simulink model "GolfSwing3D_KineticallyDrivenBlockCountStrip"  (R2024b)
settings: Solver=VariableStepAuto  StartTime=0.0  StopTime=StopTime  MaxStep=0.001  RelTol=1e-3
model workspace: external: MAT-File 3DModelInputs.mat (data not in the file)
undefined symbols (not defined in the file or in its folder): GripStrength, KillswitchFinalValue, KillswitchInitialValue, KillswitchStepTime, LeftLowerArmLength, PlaneTilt, RightLowerArmLength, UpperTorsoLength, X, Y, Z
libraries: nesl_utility x361, sm_lib x136, matrix_library x11, fl_lib x2, simulink x1
(part 11 of 13)

== matlab function GolfSwing3D_KineticallyDrivenBlockCountStrip/LScap Input Function/LScap Torque ==
  data: Time input; Killswitch input; JointTorqueLScapX output; LScapInputXA parameter; LScapInputYA parameter; LScapInputXB parameter; LScapInputYB parameter; LScapPositionSetpointX parameter; GlobalGain parameter; LScapConstantX parameter; JointTorqueLScapY output; LScapPositionInputX output; LScapPositionInputY output; LScapVelocityInputX output; LScapConstantY parameter; LScapTimeGainX parameter; LScapTimeGainY parameter; LScapInputXC parameter; LScapInputYC parameter; LScapPositionGainX parameter; LScapPositionGainY parameter; TargetLScapPositionX parameter; ModelingMode parameter; GlobalPCGain parameter; GlobalVCGain parameter; DampeningGlobalGain parameter; TargetImpactTime parameter; LScapAoX parameter; LScapAoY parameter; KinematicMode parameter; LScapDampeningX parameter; LScapDampeningY parameter; LScapPositionSetpointY parameter; LScapStartPositionX parameter; LScapStartPositionY parameter; LScapStartVelocityX parameter; LScapStartVelocityY parameter; LScapVCGainX parameter; LScapVCGainY parameter; LScapVelocityInputY output; LScapAccelerationInputX output; LScapAccelerationInputY output; LScapPCGainX parameter; LScapPCGainY parameter; LScapPositionX input; LScapPositionY input; LScapVelocityX input; LScapVelocityY input; ZVCFLScapTorqueX parameter; ZVCFLScapTorqueY parameter; TargetLScapPositionY parameter; TargetLScapVelocityX parameter; TargetLScapVelocityY parameter; LScapAfX parameter; LScapAfY parameter; LScapInputXD parameter; LScapInputXE parameter; LScapInputXF parameter; LScapInputXG parameter; LScapInputYD parameter; LScapInputYE parameter; LScapInputYF parameter; LScapInputYG parameter
function [JointTorqueLScapX,JointTorqueLScapY,LScapPositionInputX, LScapPositionInputY, LScapVelocityInputX,LScapVelocityInputY,LScapAccelerationInputX,LScapAccelerationInputY] = fcn(Time,Killswitch, LScapInputXA,LScapInputYA, LScapInputXB,LScapInputYB, LScapPositionSetpointX,GlobalGain,...
    LScapConstantX, LScapConstantY, LScapTimeGainX, LScapTimeGainY,...
    LScapInputXC, LScapInputYC, LScapPositionGainX, LScapPositionGainY,...
    TargetLScapPositionX, ModelingMode,GlobalPCGain, GlobalVCGain,DampeningGlobalGain,TargetImpactTime,LScapAoX, LScapAoY, KinematicMode, LScapDampeningX, LScapDampeningY, LScapPositionSetpointY, LScapStartPositionX,...
    LScapStartPositionY, LScapStartVelocityX, LScapStartVelocityY, LScapVCGainX,...
    LScapVCGainY, LScapPCGainX, LScapPCGainY, LScapPositionX, LScapPositionY, LScapVelocityX,...
    LScapVelocityY, ZVCFLScapTorqueX, ZVCFLScapTorqueY, TargetLScapPositionY, TargetLScapVelocityX,...
    TargetLScapVelocityY,LScapAfX, LScapAfY,LScapInputXD, LScapInputXE, LScapInputXF, LScapInputXG,...
LScapInputYD, LScapInputYE, LScapInputYF, LScapInputYG)

%Tau=Time/TargetImpactTime;
t=Time;

% %%%%%%%%%%%%%%%%%%%%%%%%%%%%%%%%%%%%%%%%%%%
% % Kinetic Input Selection and Calculation
% %%%%%%%%%%%%%%%%%%%%%%%%%%%%%%%%%%%%%%%%%%%

if ModelingMode==0
    % Values are all set to zero.
    JointTorqueLScapX=0;
    JointTorqueLScapY=0;
elseif ModelingMode==1
    % Control based strategy. Values are based on difference in value
    % between the current state and desired state.
    % LScap Joint Rotational Deltas
    DeltaLScapPositionX=LScapPositionX-TargetLScapPositionX;
    DeltaLScapPositionY=LScapPositionY-TargetLScapPositionY;
    DeltaLScapVelocityX=LScapVelocityX-TargetLScapVelocityX;
    DeltaLScapVelocityY=LScapVelocityY-TargetLScapVelocityY;
    % Control Based Strategy
    JointTorqueLScapX=DeltaLScapPositionX*LScapPCGainX*GlobalPCGain-DeltaLScapVelocityX*LScapVCGainX*GlobalVCGain-DampeningGlobalGain*LScapDampeningX*LScapVelocityX;
    JointTorqueLScapY=DeltaLScapPositionY*LScapPCGainY*GlobalPCGain-DeltaLScapVelocityY*LScapVCGainY*GlobalVCGain-DampeningGlobalGain*LScapDampeningY*LScapVelocityY;
elseif ModelingMode==2
    % Forward Dynamics Based Strategy. Values are computed based on a
    % polynomial and a combination of dampening and position gained
    % factors.
    JointTorqueLScapX=Killswitch*GlobalGain*(LScapConstantX+LScapTimeGainX*Time-LScapPositionGainX*(LScapPositionX-LScapPositionSetpointX)...
    -LScapDampeningX*LScapVelocityX);
    JointTorqueLScapY=Killswitch*GlobalGain*(LScapConstantY+LScapTimeGainY*Time-LScapPositionGainY*(LScapPositionY-LScapPositionSetpointY)...
    -LScapDampeningY*LScapVelocityY);
elseif ModelingMode==3
    JointTorqueLScapX=HexPolyInputFunction(LScapInputXA,LScapInputXB,LScapInputXC,LScapInputXD,LScapInputXE,LScapInputXF,LScapInputXG,Time)*Killswitch;
    JointTorqueLScapY=HexPolyInputFunction(LScapInputYA,LScapInputYB,LScapInputYC,LScapInputYD,LScapInputYE,LScapInputYF,LScapInputYG,Time)*Killswitch; 
else
    %ZVCF Based Joint Torques. Values are pulled from model workspace and
    %held constant.
    JointTorqueLScapX=ZVCFLScapTorqueX;
    JointTorqueLScapY=ZVCFLScapTorqueY;
end

% %%%%%%%%%%%%%%%%%%%%%%%%%%%%%%%%%%%%%%%%%%%
% % Kinematic Input Selection and Calculation
% %%%%%%%%%%%%%%%%%%%%%%%%%%%%%%%%%%%%%%%%%%%

if KinematicMode==0
    % All kinematic values set to zero.
    LScapPositionInputX=0;
    LScapPositionInputY=0;
    LScapVelocityInputX=0;
    LScapVelocityInputY=0;
    LScapAccelerationInputX=0;
    LScapAccelerationInputY=0;
elseif KinematicMode==1
    % 1st Order Acceleration, 2nd Order Velocity, 3rd Order Position Solution
    PTX=TargetLScapPositionX;       
    VTX=TargetLScapVelocityX;
    PTY=TargetLScapPositionY;
    VTY=TargetLScapVelocityY;
    % Define Starting Position and Velocity
    PIX=LScapStartPositionX;
    VIX=LScapStartVelocityX;
    PIY=LScapStartPositionY;
    VIY=LScapStartVelocityY;
    AX=3*((VTX+VIX)*TargetImpactTime-2*(PTX-PIX))/TargetImpactTime^3;         % Constant in position equation
    BX=-2*((VTX+2*VIX)*TargetImpactTime-3*(PTX-PIX))/TargetImpactTime^2;         % Constant in position equation
    CX=VIX;         % Starting Velocity at Time Zero
    DX=PIX;         % Starting Position at Time Zero
    AY=3*((VTY+VIY)*TargetImpactTime-2*(PTY-PIY))/TargetImpactTime^3;         % Constant in position equation
    BY=-2*((VTY+2*VIY)*TargetImpactTime-3*(PTY-PIY))/TargetImpactTime^2;         % Constant in position equation
    CY=VIY;         % Starting Velocity at Time Zero
    DY=PIY;         % Starting Position at Time Zero
    % Equation for position as a function of time
    LScapPositionInputX=AX*Time^3/3+BX*Time^2/2+CX*Time+DX;
    LScapPositionInputY=AY*Time^3/3+BY*Time^2/2+CY*Time+DY;
    LScapVelocityInputX=AX*Time^2+BX*Time+CX;
    LScapVelocityInputY=AY*Time^2+BY*Time+CY;
    LScapAccelerationInputX=2*AX*Time+BX;
    LScapAccelerationInputY=2*AY*Time+BY;
elseif KinematicMode==2
    % 2nd Order Acceleration, 3rd Order Velocity, 4th Order Position Solution
    Tt=TargetImpactTime;
    t=Time;
    PoX=LScapStartPositionX;
    PoY=LScapStartPositionY;
    VoX=LScapStartVelocityX;
    VoY=LScapStartVelocityY;
    PfX=TargetLScapPositionX;
    PfY=TargetLScapPositionY;
    VfX=TargetLScapVelocityX;
    VfY=TargetLScapVelocityY;
    AoX=LScapAoX;
    AoY=LScapAoY;
    LScapPositionInputX=PoX + VoX*t + (AoX*t^2)/2 - (t^3*(4*PoX - 4*PfX + Tt*VfX + 3*Tt*VoX + AoX*Tt^2))/Tt^3 + (t^4*(6*PoX - 6*PfX + 2*Tt*VfX + 4*Tt*VoX + AoX*Tt^2))/(2*Tt^4);
    LScapPositionInputY=PoY + VoY*t + (AoY*t^2)/2 - (t^3*(4*PoY - 4*PfY + Tt*VfY + 3*Tt*VoY + AoY*Tt^2))/Tt^3 + (t^4*(6*PoY - 6*PfY + 2*Tt*VfY + 4*Tt*VoY + AoY*Tt^2))/(2*Tt^4);
    LScapVelocityInputX=VoX + AoX*t - (3*t^2*(4*PoX - 4*PfX + Tt*VfX + 3*Tt*VoX + AoX*Tt^2))/Tt^3 + (2*t^3*(6*PoX - 6*PfX + 2*Tt*VfX + 4*Tt*VoX + AoX*Tt^2))/Tt^4;
    LScapVelocityInputY=VoY + AoY*t - (3*t^2*(4*PoY - 4*PfY + Tt*VfY + 3*Tt*VoY + AoY*Tt^2))/Tt^3 + (2*t^3*(6*PoY - 6*PfY + 2*Tt*VfY + 4*Tt*VoY + AoY*Tt^2))/Tt^4;
    LScapAccelerationInputX=AoX + (6*t^2*(6*PoX - 6*PfX + 2*Tt*VfX + 4*Tt*VoX + AoX*Tt^2))/Tt^4 - (6*t*(4*PoX - 4*PfX + Tt*VfX + 3*Tt*VoX + AoX*Tt^2))/Tt^3;
    LScapAccelerationInputY=AoY + (6*t^2*(6*PoY - 6*PfY + 2*Tt*VfY + 4*Tt*VoY + AoY*Tt^2))/Tt^4 - (6*t*(4*PoY - 4*PfY + Tt*VfY + 3*Tt*VoY + AoY*Tt^2))/Tt^3;
else
    % 3rd Order Acceleration, 4th Order Velocity, 5th Order Position Solution
    Tt=TargetImpactTime;
    t=Time;
    PoX=LScapStartPositionX;
    PoY=LScapStartPositionY;
    VoX=LScapStartVelocityX;
    VoY=LScapStartVelocityY;
    PfX=TargetLScapPositionX;
    PfY=TargetLScapPositionY;
    VfX=TargetLScapVelocityX;
    VfY=TargetLScapVelocityY;
    AoX=LScapAoX;
    AoY=LScapAoY;
    AfX=LScapAfX;
    AfY=LScapAfY;
    LScapPositionInputX=PoX+VoX*t+(AoX*t^2)/2-(t^5*(12*PoX-12*PfX+6*Tt*VfX+6*Tt*VoX-AfX*Tt^2+AoX*Tt^2))/(2*Tt^5)-(t^3*(20*PoX-20*PfX+8*Tt*VfX+12*Tt*VoX-AfX*Tt^2+3*AoX*Tt^2))/(2*Tt^3)+(t^4*(30*PoX-30*PfX+14*Tt*VfX+16*Tt*VoX-2*AfX*Tt^2+3*AoX*Tt^2))/(2*Tt^4);
    LScapPositionInputY=PoY+VoY*t+(AoY*t^2)/2-(t^5*(12*PoY-12*PfY+6*Tt*VfY+6*Tt*VoY-AfY*Tt^2+AoY*Tt^2))/(2*Tt^5)-(t^3*(20*PoY-20*PfY+8*Tt*VfY+12*Tt*VoY-AfY*Tt^2+3*AoY*Tt^2))/(2*Tt^3)+(t^4*(30*PoY-30*PfY+14*Tt*VfY+16*Tt*VoY-2*AfY*Tt^2+3*AoY*Tt^2))/(2*Tt^4);  
    LScapVelocityInputX=VoX+AoX*t-(5*t^4*(12*PoX-12*PfX+6*Tt*VfX+6*Tt*VoX-AfX*Tt^2+AoX*Tt^2))/(2*Tt^5)-(3*t^2*(20*PoX-20*PfX+8*Tt*VfX+12*Tt*VoX-AfX*Tt^2+3*AoX*Tt^2))/(2*Tt^3)+(2*t^3*(30*PoX-30*PfX+14*Tt*VfX+16*Tt*VoX-2*AfX*Tt^2+3*AoX*Tt^2))/Tt^4;
    LScapVelocityInputY=VoY+AoY*t-(5*t^4*(12*PoY-12*PfY+6*Tt*VfY+6*Tt*VoY-AfY*Tt^2+AoY*Tt^2))/(2*Tt^5)-(3*t^2*(20*PoY-20*PfY+8*Tt*VfY+12*Tt*VoY-AfY*Tt^2+3*AoY*Tt^2))/(2*Tt^3)+(2*t^3*(30*PoY-30*PfY+14*Tt*VfY+16*Tt*VoY-2*AfY*Tt^2+3*AoY*Tt^2))/Tt^4;
    LScapAccelerationInputX=AoX-(3*t*(20*PoX-20*PfX+8*Tt*VfX+12*Tt*VoX-AfX*Tt^2+3*AoX*Tt^2))/Tt^3-(10*t^3*(12*PoX-12*PfX+6*Tt*VfX+6*Tt*VoX-AfX*Tt^2+AoX*Tt^2))/Tt^5+(6*t^2*(30*PoX-30*PfX+14*Tt*VfX+16*Tt*VoX-2*AfX*Tt^2+3*AoX*Tt^2))/Tt^4;
    LScapAccelerationInputY=AoY-(3*t*(20*PoY-20*PfY+8*Tt*VfY+12*Tt*VoY-AfY*Tt^2+3*AoY*Tt^2))/Tt^3-(10*t^3*(12*PoY-12*PfY+6*Tt*VfY+6*Tt*VoY-AfY*Tt^2+AoY*Tt^2))/Tt^5+(6*t^2*(30*PoY-30*PfY+14*Tt*VfY+16*Tt*VoY-2*AfY*Tt^2+3*AoY*Tt^2))/Tt^4;
end

% Calculate Higher Order Derivatives of the Position Outputs
LScapJerkX=gradient(LScapAccelerationInputX,t);
LScapJerkY=gradient(LScapAccelerationInputY,t);
LScapSnapX=gradient(LScapJerkX,t);
LScapSnapY=gradient(LScapJerkY,t);
LScapCrackleX=gradient(LScapSnapX,t);
LScapCrackleY=gradient(LScapSnapY,t);
LScapPopX=gradient(LScapCrackleX,t);
LScapPopY=gradient(LScapCrackleY,t);

== matlab function GolfSwing3D_KineticallyDrivenBlockCountStrip/RScap Input Function/RScap Torque ==
  data: Time input; Killswitch input; JointTorqueRScapX output; RScapInputXA parameter; RScapInputYA parameter; RScapInputXB parameter; RScapInputYB parameter; RScapPositionSetpointX parameter; GlobalGain parameter; RScapConstantX parameter; JointTorqueRScapY output; RScapConstantY parameter; RScapTimeGainX parameter; RScapTimeGainY parameter; RScapInputXC parameter; RScapInputYC parameter; RScapPositionGainX parameter; RScapPositionGainY parameter; TargetRScapPositionX parameter; ModelingMode parameter; GlobalPCGain parameter; GlobalVCGain parameter; DampeningGlobalGain parameter; TargetImpactTime parameter; KinematicMode parameter; RScapPositionSetpointY parameter; RScapStartPositionX parameter; RScapStartPositionY parameter; RScapVCGainX parameter; RScapVCGainY parameter; RScapPCGainX parameter; RScapPCGainY parameter; RScapPositionInputX output; RScapPositionInputY output; RScapVelocityInputX output; RScapVelocityInputY output; RScapAccelerationInputX output; RScapAccelerationInputY output; ZVCFRScapTorqueX parameter; ZVCFRScapTorqueY parameter; TargetRScapPositionY parameter; TargetRScapVelocityX parameter; TargetRScapVelocityY parameter; RScapAoX parameter; RScapAoY parameter; RScapDampeningX parameter; RScapDampeningY parameter; RScapPositionX input; RScapPositionY input; RScapVelocityX input; RScapVelocityY input; RScapStartVelocityX parameter; RScapStartVelocityY parameter; RScapAfX parameter; RScapAfY parameter; RScapInputXD parameter; RScapInputXE parameter; RScapInputXF parameter; RScapInputXG parameter; RScapInputYD parameter; RScapInputYE parameter; RScapInputYF parameter; RScapInputYG parameter
function [JointTorqueRScapX,JointTorqueRScapY,RScapPositionInputX,...
    RScapPositionInputY, RScapVelocityInputX,RScapVelocityInputY,...
    RScapAccelerationInputX,RScapAccelerationInputY] = fcn(Time,Killswitch,...
    RScapInputXA,RScapInputYA, RScapInputXB,RScapInputYB, RScapPositionSetpointX,GlobalGain,...
    RScapConstantX, RScapConstantY, RScapTimeGainX, RScapTimeGainY,...
    RScapInputXC, RScapInputYC, RScapPositionGainX, RScapPositionGainY,...
    TargetRScapPositionX, ModelingMode,GlobalPCGain, GlobalVCGain,DampeningGlobalGain,...
    TargetImpactTime,KinematicMode, RScapPositionSetpointY, RScapStartPositionX,...
    RScapStartPositionY, RScapVCGainX,RScapVCGainY, RScapPCGainX, RScapPCGainY,...
    ZVCFRScapTorqueX, ZVCFRScapTorqueY, ...
    TargetRScapPositionY, TargetRScapVelocityX, TargetRScapVelocityY,...
    RScapAoX, RScapAoY, RScapDampeningX, RScapDampeningY, RScapPositionX,...
    RScapPositionY, RScapVelocityX, RScapVelocityY, RScapStartVelocityX, RScapStartVelocityY,...
    RScapAfX, RScapAfY,RScapInputXD, RScapInputXE, RScapInputXF, RScapInputXG,...
RScapInputYD, RScapInputYE, RScapInputYF, RScapInputYG)

%Tau=Time/TargetImpactTime;
t=Time;

% %%%%%%%%%%%%%%%%%%%%%%%%%%%%%%%%%%%%%%%%%%%
% % Kinetic Input Selection and Calculation
% %%%%%%%%%%%%%%%%%%%%%%%%%%%%%%%%%%%%%%%%%%%

if ModelingMode==0
    % Values are all set to zero.
    JointTorqueRScapX=0;
    JointTorqueRScapY=0;
elseif ModelingMode==1
    % Control based strategy. Values are based on difference in value
    % between the current state and desired state.
    % RScap Joint Rotational Deltas
    DeltaRScapPositionX=RScapPositionX-TargetRScapPositionX;
    DeltaRScapPositionY=RScapPositionY-TargetRScapPositionY;
    DeltaRScapVelocityX=RScapVelocityX-TargetRScapVelocityX;
    DeltaRScapVelocityY=RScapVelocityY-TargetRScapVelocityY;
    % Control Based Strategy
    JointTorqueRScapX=DeltaRScapPositionX*RScapPCGainX*GlobalPCGain-DeltaRScapVelocityX*RScapVCGainX*GlobalVCGain-DampeningGlobalGain*RScapDampeningX*RScapVelocityX;
    JointTorqueRScapY=DeltaRScapPositionY*RScapPCGainY*GlobalPCGain-DeltaRScapVelocityY*RScapVCGainY*GlobalVCGain-DampeningGlobalGain*RScapDampeningY*RScapVelocityY;
elseif ModelingMode==2
    % Forward Dynamics Based Strategy. Values are computed based on a
    % polynomial and a combination of dampening and position gained
    % factors.
    JointTorqueRScapX=Killswitch*GlobalGain*(RScapConstantX+RScapTimeGainX*Time-RScapPositionGainX*(RScapPositionX-RScapPositionSetpointX)...
    -RScapDampeningX*RScapVelocityX);
    JointTorqueRScapY=Killswitch*GlobalGain*(RScapConstantY+RScapTimeGainY*Time-RScapPositionGainY*(RScapPositionY-RScapPositionSetpointY)...
    -RScapDampeningY*RScapVelocityY);
elseif ModelingMode==3
    JointTorqueRScapX=HexPolyInputFunction(RScapInputXA,RScapInputXB,RScapInputXC,RScapInputXD,RScapInputXE,RScapInputXF,RScapInputXG,Time)*Killswitch;
    JointTorqueRScapY=HexPolyInputFunction(RScapInputYA,RScapInputYB,RScapInputYC,RScapInputYD,RScapInputYE,RScapInputYF,RScapInputYG,Time)*Killswitch;  
else
    %ZVCF Based Joint Torques. Values are pulled from model workspace and
    %held constant.
    JointTorqueRScapX=ZVCFRScapTorqueX;
    JointTorqueRScapY=ZVCFRScapTorqueY;
end

% %%%%%%%%%%%%%%%%%%%%%%%%%%%%%%%%%%%%%%%%%%%
% % Kinematic Input Selection and Calculation
% %%%%%%%%%%%%%%%%%%%%%%%%%%%%%%%%%%%%%%%%%%%

if KinematicMode==0
    % All kinematic values set to zero.
    RScapPositionInputX=0;
    RScapPositionInputY=0;
    RScapVelocityInputX=0;
    RScapVelocityInputY=0;
    RScapAccelerationInputX=0;
    RScapAccelerationInputY=0;
elseif KinematicMode==1
    % 1st Order Acceleration, 2nd Order Velocity, 3rd Order Position Solution
    PTX=TargetRScapPositionX;       
    VTX=TargetRScapVelocityX;
    PTY=TargetRScapPositionY;
    VTY=TargetRScapVelocityY;
    % Define Starting Position and Velocity
    PIX=RScapStartPositionX;
    VIX=RScapStartVelocityX;
    PIY=RScapStartPositionY;
    VIY=RScapStartVelocityY;
    AX=3*((VTX+VIX)*TargetImpactTime-2*(PTX-PIX))/TargetImpactTime^3;         % Constant in position equation
    BX=-2*((VTX+2*VIX)*TargetImpactTime-3*(PTX-PIX))/TargetImpactTime^2;         % Constant in position equation
    CX=VIX;         % Starting Velocity at Time Zero
    DX=PIX;         % Starting Position at Time Zero
    AY=3*((VTY+VIY)*TargetImpactTime-2*(PTY-PIY))/TargetImpactTime^3;         % Constant in position equation
    BY=-2*((VTY+2*VIY)*TargetImpactTime-3*(PTY-PIY))/TargetImpactTime^2;         % Constant in position equation
    CY=VIY;         % Starting Velocity at Time Zero
    DY=PIY;         % Starting Position at Time Zero
    % Equation for position as a function of time
    RScapPositionInputX=AX*Time^3/3+BX*Time^2/2+CX*Time+DX;
    RScapPositionInputY=AY*Time^3/3+BY*Time^2/2+CY*Time+DY;
    RScapVelocityInputX=AX*Time^2+BX*Time+CX;
    RScapVelocityInputY=AY*Time^2+BY*Time+CY;
    RScapAccelerationInputX=2*AX*Time+BX;
    RScapAccelerationInputY=2*AY*Time+BY;
elseif KinematicMode==2
    % 2nd Order Acceleration, 3rd Order Velocity, 4th Order Position Solution
    Tt=TargetImpactTime;
    t=Time;
    PoX=RScapStartPositionX;
    PoY=RScapStartPositionY;
    VoX=RScapStartVelocityX;
    VoY=RScapStartVelocityY;
    PfX=TargetRScapPositionX;
    PfY=TargetRScapPositionY;
    VfX=TargetRScapVelocityX;
    VfY=TargetRScapVelocityY;
    AoX=RScapAoX;
    AoY=RScapAoY;
    RScapPositionInputX=PoX + VoX*t + (AoX*t^2)/2 - (t^3*(4*PoX - 4*PfX + Tt*VfX + 3*Tt*VoX + AoX*Tt^2))/Tt^3 + (t^4*(6*PoX - 6*PfX + 2*Tt*VfX + 4*Tt*VoX + AoX*Tt^2))/(2*Tt^4);
    RScapPositionInputY=PoY + VoY*t + (AoY*t^2)/2 - (t^3*(4*PoY - 4*PfY + Tt*VfY + 3*Tt*VoY + AoY*Tt^2))/Tt^3 + (t^4*(6*PoY - 6*PfY + 2*Tt*VfY + 4*Tt*VoY + AoY*Tt^2))/(2*Tt^4);
    RScapVelocityInputX=VoX + AoX*t - (3*t^2*(4*PoX - 4*PfX + Tt*VfX + 3*Tt*VoX + AoX*Tt^2))/Tt^3 + (2*t^3*(6*PoX - 6*PfX + 2*Tt*VfX + 4*Tt*VoX + AoX*Tt^2))/Tt^4;
    RScapVelocityInputY=VoY + AoY*t - (3*t^2*(4*PoY - 4*PfY + Tt*VfY + 3*Tt*VoY + AoY*Tt^2))/Tt^3 + (2*t^3*(6*PoY - 6*PfY + 2*Tt*VfY + 4*Tt*VoY + AoY*Tt^2))/Tt^4;
    RScapAccelerationInputX=AoX + (6*t^2*(6*PoX - 6*PfX + 2*Tt*VfX + 4*Tt*VoX + AoX*Tt^2))/Tt^4 - (6*t*(4*PoX - 4*PfX + Tt*VfX + 3*Tt*VoX + AoX*Tt^2))/Tt^3;
    RScapAccelerationInputY=AoY + (6*t^2*(6*PoY - 6*PfY + 2*Tt*VfY + 4*Tt*VoY + AoY*Tt^2))/Tt^4 - (6*t*(4*PoY - 4*PfY + Tt*VfY + 3*Tt*VoY + AoY*Tt^2))/Tt^3;
else
    % 3rd Order Acceleration, 4th Order Velocity, 5th Order Position Solution
    Tt=TargetImpactTime;
    t=Time;
    PoX=RScapStartPositionX;
    PoY=RScapStartPositionY;
    VoX=RScapStartVelocityX;
    VoY=RScapStartVelocityY;
    PfX=TargetRScapPositionX;
    PfY=TargetRScapPositionY;
    VfX=TargetRScapVelocityX;
    VfY=TargetRScapVelocityY;
    AoX=RScapAoX;
    AoY=RScapAoY;
    AfX=RScapAfX;
    AfY=RScapAfY;
    RScapPositionInputX=PoX+VoX*t+(AoX*t^2)/2-(t^5*(12*PoX-12*PfX+6*Tt*VfX+6*Tt*VoX-AfX*Tt^2+AoX*Tt^2))/(2*Tt^5)-(t^3*(20*PoX-20*PfX+8*Tt*VfX+12*Tt*VoX-AfX*Tt^2+3*AoX*Tt^2))/(2*Tt^3)+(t^4*(30*PoX-30*PfX+14*Tt*VfX+16*Tt*VoX-2*AfX*Tt^2+3*AoX*Tt^2))/(2*Tt^4);
    RScapPositionInputY=PoY+VoY*t+(AoY*t^2)/2-(t^5*(12*PoY-12*PfY+6*Tt*VfY+6*Tt*VoY-AfY*Tt^2+AoY*Tt^2))/(2*Tt^5)-(t^3*(20*PoY-20*PfY+8*Tt*VfY+12*Tt*VoY-AfY*Tt^2+3*AoY*Tt^2))/(2*Tt^3)+(t^4*(30*PoY-30*PfY+14*Tt*VfY+16*Tt*VoY-2*AfY*Tt^2+3*AoY*Tt^2))/(2*Tt^4);  
    RScapVelocityInputX=VoX+AoX*t-(5*t^4*(12*PoX-12*PfX+6*Tt*VfX+6*Tt*VoX-AfX*Tt^2+AoX*Tt^2))/(2*Tt^5)-(3*t^2*(20*PoX-20*PfX+8*Tt*VfX+12*Tt*VoX-AfX*Tt^2+3*AoX*Tt^2))/(2*Tt^3)+(2*t^3*(30*PoX-30*PfX+14*Tt*VfX+16*Tt*VoX-2*AfX*Tt^2+3*AoX*Tt^2))/Tt^4;
    RScapVelocityInputY=VoY+AoY*t-(5*t^4*(12*PoY-12*PfY+6*Tt*VfY+6*Tt*VoY-AfY*Tt^2+AoY*Tt^2))/(2*Tt^5)-(3*t^2*(20*PoY-20*PfY+8*Tt*VfY+12*Tt*VoY-AfY*Tt^2+3*AoY*Tt^2))/(2*Tt^3)+(2*t^3*(30*PoY-30*PfY+14*Tt*VfY+16*Tt*VoY-2*AfY*Tt^2+3*AoY*Tt^2))/Tt^4;
    RScapAccelerationInputX=AoX-(3*t*(20*PoX-20*PfX+8*Tt*VfX+12*Tt*VoX-AfX*Tt^2+3*AoX*Tt^2))/Tt^3-(10*t^3*(12*PoX-12*PfX+6*Tt*VfX+6*Tt*VoX-AfX*Tt^2+AoX*Tt^2))/Tt^5+(6*t^2*(30*PoX-30*PfX+14*Tt*VfX+16*Tt*VoX-2*AfX*Tt^2+3*AoX*Tt^2))/Tt^4;
    RScapAccelerationInputY=AoY-(3*t*(20*PoY-20*PfY+8*Tt*VfY+12*Tt*VoY-AfY*Tt^2+3*AoY*Tt^2))/Tt^3-(10*t^3*(12*PoY-12*PfY+6*Tt*VfY+6*Tt*VoY-AfY*Tt^2+AoY*Tt^2))/Tt^5+(6*t^2*(30*PoY-30*PfY+14*Tt*VfY+16*Tt*VoY-2*AfY*Tt^2+3*AoY*Tt^2))/Tt^4;
end

% Calculate Higher Order Derivatives of the Position Outputs
RScapJerkX=gradient(RScapAccelerationInputX,t);
RScapJerkY=gradient(RScapAccelerationInputY,t);
RScapSnapX=gradient(RScapJerkX,t);
RScapSnapY=gradient(RScapJerkY,t);
RScapCrackleX=gradient(RScapSnapX,t);
RScapCrackleY=gradient(RScapSnapY,t);
RScapPopX=gradient(RScapCrackleX,t);
RScapPopY=gradient(RScapCrackleY,t);

== matlab function GolfSwing3D_KineticallyDrivenBlockCountStrip/Left Hand/LW Unit Vector ==
  data: LWv input; LWSpeed output; LWvx input; LWvy input; LWvz input; LWuvx output; LWuvy output; LWuvz output
function [LWSpeed,LWuvx,LWuvy,LWuvz]  = fcn(LWv,LWvx,LWvy,LWvz)

LWSpeed=norm(LWv);
LWuvx=LWvx/LWSpeed;
LWuvy=LWvy/LWSpeed;
LWuvz=LWvz/LWSpeed;

== matlab function GolfSwing3D_KineticallyDrivenBlockCountStrip/Midpoint/MP Unit Vector ==
  data: MPv input; MidHandSpeed output; MPvx input; MPvy input; MPvz input; MPuvx output; MPuvy output; MPuvz output
function [MidHandSpeed,MPuvx,MPuvy,MPuvz]  = fcn(MPv,MPvx,MPvy,MPvz)

MidHandSpeed=norm(MPv);
MPuvx=MPvx/MidHandSpeed;
MPuvy=MPvy/MidHandSpeed;
MPuvz=MPvz/MidHandSpeed;

== matlab function GolfSwing3D_KineticallyDrivenBlockCountStrip/LW Input Function/Left Wrist Torque ==
  data: Time input; Killswitch input; JointTorqueLWX output; LWInputXA parameter; LWInputYA parameter; LWInputXB parameter; LWInputYB parameter; LWPositionSetpointX parameter; GlobalGain parameter; JointTorqueLWY output; LWConstantX parameter; LWConstantY parameter; LWTimeGainX parameter; LWTimeGainY parameter; LWInputXC parameter; LWInputYC parameter; LWPositionGainX parameter; LWPositionGainY parameter; TargetLWPositionX parameter; ModelingMode parameter; GlobalPCGain parameter; GlobalVCGain parameter; DampeningGlobalGain parameter; TargetImpactTime parameter; KinematicMode parameter; LWPositionSetpointY parameter; LWStartPositionX parameter; LWStartPositionY parameter; LWStartVelocityX parameter; LWStartVelocityY parameter; LWVCGainX parameter; LWVCGainY parameter; LWPCGainX parameter; LWPCGainY parameter; LWPositionInputX output; LWPositionInputY output; LWVelocityInputX output; LWVelocityInputY output; LWAccelerationInputX output; LWAccelerationInputY output; ZVCFLWTorqueX parameter; ZVCFLWTorqueY parameter; LWAoX parameter; LWAoY parameter; LWDampeningX parameter; LWDampeningY parameter; TargetLWPositionY parameter; TargetLWVelocityX parameter; TargetLWVelocityY parameter; LWPositionX input; LWPositionY input; LWVelocityX input; LWVelocityY input; LWAfX parameter; LWAfY parameter; LWInputXD parameter; LWInputXE parameter; LWInputXF parameter; LWInputXG parameter; LWInputYD parameter; LWInputYE parameter; LWInputYF parameter; LWInputYG parameter; LWLocaltoGlobalR input; LWTorqueGlobal input; LWJointTorqueInputGlobal output; LWConstraintTorque output
function [JointTorqueLWX,JointTorqueLWY,LWPositionInputX, LWPositionInputY,...
    LWVelocityInputX,LWVelocityInputY,LWAccelerationInputX,LWAccelerationInputY,...
    LWJointTorqueInputGlobal,LWConstraintTorque]...
    = fcn(Time,Killswitch, LWInputXA,LWInputYA, LWInputXB,LWInputYB, LWPositionSetpointX,GlobalGain,...
    LWConstantX, LWConstantY, LWTimeGainX, LWTimeGainY,...
    LWInputXC, LWInputYC, LWPositionGainX, LWPositionGainY,...
    TargetLWPositionX, ModelingMode,GlobalPCGain, GlobalVCGain,DampeningGlobalGain,TargetImpactTime,KinematicMode, LWPositionSetpointY, LWStartPositionX,...
    LWStartPositionY, LWStartVelocityX, LWStartVelocityY, LWVCGainX,...
    LWVCGainY, LWPCGainX, LWPCGainY, ZVCFLWTorqueX, ZVCFLWTorqueY, LWAoX,...
    LWAoY, LWDampeningX, LWDampeningY, TargetLWPositionY, TargetLWVelocityX,...
    TargetLWVelocityY, LWPositionX, LWPositionY, LWVelocityX, LWVelocityY,...
    LWAfX, LWAfY,LWInputXD, LWInputXE, LWInputXF, LWInputXG, LWInputYD, LWInputYE, LWInputYF, LWInputYG,LWLocaltoGlobalR,LWTorqueGlobal)

%Tau=Time/TargetImpactTime;
t=Time;

% %%%%%%%%%%%%%%%%%%%%%%%%%%%%%%%%%%%%%%%%%%%
% % Kinetic Input Selection and Calculation
% %%%%%%%%%%%%%%%%%%%%%%%%%%%%%%%%%%%%%%%%%%%

if ModelingMode==0
    % Values are all set to zero.
    JointTorqueLWX=0;
    JointTorqueLWY=0;
elseif ModelingMode==1
    % Control based strategy. Values are based on difference in value
    % between the current state and desired state.
    % LW Joint Rotational Deltas
    DeltaLWPositionX=LWPositionX-TargetLWPositionX;
    DeltaLWPositionY=LWPositionY-TargetLWPositionY;
    DeltaLWVelocityX=LWVelocityX-TargetLWVelocityX;
    DeltaLWVelocityY=LWVelocityY-TargetLWVelocityY;
    % Control Based Strategy
    JointTorqueLWX=DeltaLWPositionX*LWPCGainX*GlobalPCGain-DeltaLWVelocityX*LWVCGainX*GlobalVCGain-DampeningGlobalGain*LWDampeningX*LWVelocityX;
    JointTorqueLWY=DeltaLWPositionY*LWPCGainY*GlobalPCGain-DeltaLWVelocityY*LWVCGainY*GlobalVCGain-DampeningGlobalGain*LWDampeningY*LWVelocityY;
elseif ModelingMode==2
    % Forward Dynamics Based Strategy. Values are computed based on a
    % polynomial and a combination of dampening and position gained
    % factors.
    JointTorqueLWX=Killswitch*GlobalGain*(LWConstantX+LWTimeGainX*Time-LWPositionGainX*(LWPositionX-LWPositionSetpointX)...
    -LWDampeningX*LWVelocityX);
    JointTorqueLWY=Killswitch*GlobalGain*(LWConstantY+LWTimeGainY*Time-LWPositionGainY*(LWPositionY-LWPositionSetpointY)...
    -LWDampeningY*LWVelocityY);
elseif ModelingMode==3
    JointTorqueLWX=HexPolyInputFunction(LWInputXA,LWInputXB,LWInputXC,LWInputXD,LWInputXE,LWInputXF,LWInputXG,Time)*Killswitch;
    JointTorqueLWY=HexPolyInputFunction(LWInputYA,LWInputYB,LWInputYC,LWInputYD,LWInputYE,LWInputYF,LWInputYG,Time)*Killswitch;  
else
    %ZVCF Based Joint Torques. Values are pulled from model workspace and
    %held constant.
    JointTorqueLWX=ZVCFLWTorqueX;
    JointTorqueLWY=ZVCFLWTorqueY;
end

% Create a global vector of the joint torque inputs
LWJointTorqueInputLocal=cat(1,JointTorqueLWX,JointTorqueLWY,0);
LWJointTorqueInputGlobal=LWLocaltoGlobalR*LWJointTorqueInputLocal;
% 
% Compare total torque measured to input torques applied to see the
% constraint torque
LWConstraintTorque=LWTorqueGlobal-LWJointTorqueInputGlobal;

% %%%%%%%%%%%%%%%%%%%%%%%%%%%%%%%%%%%%%%%%%%%
% % Kinematic Input Selection and Calculation
% %%%%%%%%%%%%%%%%%%%%%%%%%%%%%%%%%%%%%%%%%%%

if KinematicMode==0
    % All kinematic values set to zero.
    LWPositionInputX=0;
    LWPositionInputY=0;
    LWVelocityInputX=0;
    LWVelocityInputY=0;
    LWAccelerationInputX=0;
    LWAccelerationInputY=0;
elseif KinematicMode==1
    % 1st Order Acceleration, 2nd Order Velocity, 3rd Order Position Solution
    PTX=TargetLWPositionX;       
    VTX=TargetLWVelocityX;
    PTY=TargetLWPositionY;
    VTY=TargetLWVelocityY;
    % Define Starting Position and Velocity
    PIX=LWStartPositionX;
    VIX=LWStartVelocityX;
    PIY=LWStartPositionY;
    VIY=LWStartVelocityY;
    AX=3*((VTX+VIX)*TargetImpactTime-2*(PTX-PIX))/TargetImpactTime^3;         % Constant in position equation
    BX=-2*((VTX+2*VIX)*TargetImpactTime-3*(PTX-PIX))/TargetImpactTime^2;         % Constant in position equation
    CX=VIX;         % Starting Velocity at Time Zero
    DX=PIX;         % Starting Position at Time Zero
    AY=3*((VTY+VIY)*TargetImpactTime-2*(PTY-PIY))/TargetImpactTime^3;         % Constant in position equation
    BY=-2*((VTY+2*VIY)*TargetImpactTime-3*(PTY-PIY))/TargetImpactTime^2;         % Constant in position equation
    CY=VIY;         % Starting Velocity at Time Zero
    DY=PIY;         % Starting Position at Time Zero
    % Equation for position as a function of time
    LWPositionInputX=AX*Time^3/3+BX*Time^2/2+CX*Time+DX;
    LWPositionInputY=AY*Time^3/3+BY*Time^2/2+CY*Time+DY;
    LWVelocityInputX=AX*Time^2+BX*Time+CX;
    LWVelocityInputY=AY*Time^2+BY*Time+CY;
    LWAccelerationInputX=2*AX*Time+BX;
    LWAccelerationInputY=2*AY*Time+BY;
elseif KinematicMode==2
    % 2nd Order Acceleration, 3rd Order Velocity, 4th Order Position Solution
    Tt=TargetImpactTime;
    t=Time;
    PoX=LWStartPositionX;
    PoY=LWStartPositionY;
    VoX=LWStartVelocityX;
    VoY=LWStartVelocityY;
    PfX=TargetLWPositionX;
    PfY=TargetLWPositionY;
    VfX=TargetLWVelocityX;
    VfY=TargetLWVelocityY;
    AoX=LWAoX;
    AoY=LWAoY;
    LWPositionInputX=PoX + VoX*t + (AoX*t^2)/2 - (t^3*(4*PoX - 4*PfX + Tt*VfX + 3*Tt*VoX + AoX*Tt^2))/Tt^3 + (t^4*(6*PoX - 6*PfX + 2*Tt*VfX + 4*Tt*VoX + AoX*Tt^2))/(2*Tt^4);
    LWPositionInputY=PoY + VoY*t + (AoY*t^2)/2 - (t^3*(4*PoY - 4*PfY + Tt*VfY + 3*Tt*VoY + AoY*Tt^2))/Tt^3 + (t^4*(6*PoY - 6*PfY + 2*Tt*VfY + 4*Tt*VoY + AoY*Tt^2))/(2*Tt^4);
    LWVelocityInputX=VoX + AoX*t - (3*t^2*(4*PoX - 4*PfX + Tt*VfX + 3*Tt*VoX + AoX*Tt^2))/Tt^3 + (2*t^3*(6*PoX - 6*PfX + 2*Tt*VfX + 4*Tt*VoX + AoX*Tt^2))/Tt^4;
    LWVelocityInputY=VoY + AoY*t - (3*t^2*(4*PoY - 4*PfY + Tt*VfY + 3*Tt*VoY + AoY*Tt^2))/Tt^3 + (2*t^3*(6*PoY - 6*PfY + 2*Tt*VfY + 4*Tt*VoY + AoY*Tt^2))/Tt^4;
    LWAccelerationInputX=AoX + (6*t^2*(6*PoX - 6*PfX + 2*Tt*VfX + 4*Tt*VoX + AoX*Tt^2))/Tt^4 - (6*t*(4*PoX - 4*PfX + Tt*VfX + 3*Tt*VoX + AoX*Tt^2))/Tt^3;
    LWAccelerationInputY=AoY + (6*t^2*(6*PoY - 6*PfY + 2*Tt*VfY + 4*Tt*VoY + AoY*Tt^2))/Tt^4 - (6*t*(4*PoY - 4*PfY + Tt*VfY + 3*Tt*VoY + AoY*Tt^2))/Tt^3;
else
    % 3rd Order Acceleration, 4th Order Velocity, 5th Order Position Solution
    Tt=TargetImpactTime;
    t=Time;
    PoX=LWStartPositionX;
    PoY=LWStartPositionY;
    VoX=LWStartVelocityX;
    VoY=LWStartVelocityY;
    PfX=TargetLWPositionX;
    PfY=TargetLWPositionY;
    VfX=TargetLWVelocityX;
    VfY=TargetLWVelocityY;
    AoX=LWAoX;
    AoY=LWAoY;
    AfX=LWAfX;
    AfY=LWAfY;
    LWPositionInputX=PoX+VoX*t+(AoX*t^2)/2-(t^5*(12*PoX-12*PfX+6*Tt*VfX+6*Tt*VoX-AfX*Tt^2+AoX*Tt^2))/(2*Tt^5)-(t^3*(20*PoX-20*PfX+8*Tt*VfX+12*Tt*VoX-AfX*Tt^2+3*AoX*Tt^2))/(2*Tt^3)+(t^4*(30*PoX-30*PfX+14*Tt*VfX+16*Tt*VoX-2*AfX*Tt^2+3*AoX*Tt^2))/(2*Tt^4);
    LWPositionInputY=PoY+VoY*t+(AoY*t^2)/2-(t^5*(12*PoY-12*PfY+6*Tt*VfY+6*Tt*VoY-AfY*Tt^2+AoY*Tt^2))/(2*Tt^5)-(t^3*(20*PoY-20*PfY+8*Tt*VfY+12*Tt*VoY-AfY*Tt^2+3*AoY*Tt^2))/(2*Tt^3)+(t^4*(30*PoY-30*PfY+14*Tt*VfY+16*Tt*VoY-2*AfY*Tt^2+3*AoY*Tt^2))/(2*Tt^4);  
    LWVelocityInputX=VoX+AoX*t-(5*t^4*(12*PoX-12*PfX+6*Tt*VfX+6*Tt*VoX-AfX*Tt^2+AoX*Tt^2))/(2*Tt^5)-(3*t^2*(20*PoX-20*PfX+8*Tt*VfX+12*Tt*VoX-AfX*Tt^2+3*AoX*Tt^2))/(2*Tt^3)+(2*t^3*(30*PoX-30*PfX+14*Tt*VfX+16*Tt*VoX-2*AfX*Tt^2+3*AoX*Tt^2))/Tt^4;
    LWVelocityInputY=VoY+AoY*t-(5*t^4*(12*PoY-12*PfY+6*Tt*VfY+6*Tt*VoY-AfY*Tt^2+AoY*Tt^2))/(2*Tt^5)-(3*t^2*(20*PoY-20*PfY+8*Tt*VfY+12*Tt*VoY-AfY*Tt^2+3*AoY*Tt^2))/(2*Tt^3)+(2*t^3*(30*PoY-30*PfY+14*Tt*VfY+16*Tt*VoY-2*AfY*Tt^2+3*AoY*Tt^2))/Tt^4;
    LWAccelerationInputX=AoX-(3*t*(20*PoX-20*PfX+8*Tt*VfX+12*Tt*VoX-AfX*Tt^2+3*AoX*Tt^2))/Tt^3-(10*t^3*(12*PoX-12*PfX+6*Tt*VfX+6*Tt*VoX-AfX*Tt^2+AoX*Tt^2))/Tt^5+(6*t^2*(30*PoX-30*PfX+14*Tt*VfX+16*Tt*VoX-2*AfX*Tt^2+3*AoX*Tt^2))/Tt^4;
    LWAccelerationInputY=AoY-(3*t*(20*PoY-20*PfY+8*Tt*VfY+12*Tt*VoY-AfY*Tt^2+3*AoY*Tt^2))/Tt^3-(10*t^3*(12*PoY-12*PfY+6*Tt*VfY+6*Tt*VoY-AfY*Tt^2+AoY*Tt^2))/Tt^5+(6*t^2*(30*PoY-30*PfY+14*Tt*VfY+16*Tt*VoY-2*AfY*Tt^2+3*AoY*Tt^2))/Tt^4;
end


% Calculate Higher Order Derivatives of the Position Outputs
LWJerkX=gradient(LWAccelerationInputX,t);
LWJerkY=gradient(LWAccelerationInputY,t);
LWSnapX=gradient(LWJerkX,t);
LWSnapY=gradient(LWJerkY,t);
LWCrackleX=gradient(LWSnapX,t);
LWCrackleY=gradient(LWSnapY,t);
LWPopX=gradient(LWCrackleX,t);
LWPopY=gradient(LWCrackleY,t);

== matlab function GolfSwing3D_KineticallyDrivenBlockCountStrip/RW Input Function/Right Wrist Torque ==
  data: Time input; Killswitch input; JointTorqueRWX output; RWInputXA parameter; RWInputYA parameter; RWInputXB parameter; RWInputYB parameter; RWPositionSetpointX parameter; GlobalGain parameter; JointTorqueRWY output; RWConstantX parameter; RWConstantY parameter; RWTimeGainX parameter; RWTimeGainY parameter; RWInputXC parameter; RWInputYC parameter; RWPositionGainX parameter; RWPositionGainY parameter; TargetRWPositionX parameter; ModelingMode parameter; GlobalPCGain parameter; GlobalVCGain parameter; DampeningGlobalGain parameter; TargetImpactTime parameter; KinematicMode parameter; RWVCGainY parameter; RWPCGainX parameter; RWPCGainY parameter; ZVCFRWTorqueX parameter; ZVCFRWTorqueY parameter; TargetRWPositionY parameter; TargetRWVelocityX parameter; TargetRWVelocityY parameter; RWAoX parameter; RWPositionInputX output; RWPositionInputY output; RWVelocityInputX output; RWVelocityInputY output; RWAccelerationInputX output; RWAccelerationInputY output; RWAoY parameter; RWDampeningX parameter; RWDampeningY parameter; RWPositionX input; RWPositionY input; RWStartPositionX parameter; RWStartPositionY parameter; RWStartVelocityX parameter; RWStartVelocityY parameter; RWVCGainX parameter; RWPositionSetpointY parameter; RWVelocityX input; RWVelocityY input; RWAfX parameter; RWAfY parameter; RWInputXD parameter; RWInputXE parameter; RWInputXF parameter; RWInputXG parameter; RWInputYD parameter; RWInputYE parameter; RWInputYF parameter; RWInputYG parameter; RWLocaltoGlobalR input; RWTorqueGlobal input; RWJointTorqueInputGlobal output; RWConstraintTorque output
function [JointTorqueRWX,JointTorqueRWY,RWPositionInputX, RWPositionInputY,...
    RWVelocityInputX,RWVelocityInputY,RWAccelerationInputX,RWAccelerationInputY,...
    RWJointTorqueInputGlobal,RWConstraintTorque]...
    = fcn(Time,Killswitch, RWInputXA,RWInputYA, RWInputXB,RWInputYB, RWPositionSetpointX,GlobalGain,...
    RWConstantX, RWConstantY, RWTimeGainX, RWTimeGainY,...
    RWInputXC, RWInputYC, RWPositionGainX, RWPositionGainY,...
    TargetRWPositionX, ModelingMode,GlobalPCGain, GlobalVCGain,...
    DampeningGlobalGain,TargetImpactTime,KinematicMode, RWVCGainY,...
    RWPCGainX, RWPCGainY, ZVCFRWTorqueX, ...
    ZVCFRWTorqueY, TargetRWPositionY, TargetRWVelocityX, TargetRWVelocityY,...
    RWAoX, RWAoY, RWDampeningX, RWDampeningY, RWPositionX, RWPositionY, RWStartPositionX,...
    RWStartPositionY, RWStartVelocityX, RWStartVelocityY, RWVCGainX,...
    RWPositionSetpointY, RWVelocityX, RWVelocityY,RWAfX, RWAfY,RWInputXD, RWInputXE, RWInputXF,...
RWInputXG, RWInputYD, RWInputYE, RWInputYF, RWInputYG,RWLocaltoGlobalR,RWTorqueGlobal)

%Tau=Time/TargetImpactTime;
t=Time;

% %%%%%%%%%%%%%%%%%%%%%%%%%%%%%%%%%%%%%%%%%%%
% % Kinetic Input Selection and Calculation
% %%%%%%%%%%%%%%%%%%%%%%%%%%%%%%%%%%%%%%%%%%%

if ModelingMode==0
    % Values are all set to zero.
    JointTorqueRWX=0;
    JointTorqueRWY=0;
elseif ModelingMode==1
    % Control based strategy. Values are based on difference in value
    % between the current state and desired state.
    % RW Joint Rotational Deltas
    DeltaRWPositionX=RWPositionX-TargetRWPositionX;
    DeltaRWPositionY=RWPositionY-TargetRWPositionY;
    DeltaRWVelocityX=RWVelocityX-TargetRWVelocityX;
    DeltaRWVelocityY=RWVelocityY-TargetRWVelocityY;
    % Control Based Strategy
    JointTorqueRWX=DeltaRWPositionX*RWPCGainX*GlobalPCGain-DeltaRWVelocityX*RWVCGainX*GlobalVCGain-DampeningGlobalGain*RWDampeningX*RWVelocityX;
    JointTorqueRWY=DeltaRWPositionY*RWPCGainY*GlobalPCGain-DeltaRWVelocityY*RWVCGainY*GlobalVCGain-DampeningGlobalGain*RWDampeningY*RWVelocityY;
elseif ModelingMode==2
    % Forward Dynamics Based Strategy. Values are computed based on a
    % polynomial and a combination of dampening and position gained
    % factors.
    JointTorqueRWX=Killswitch*GlobalGain*(RWConstantX+RWTimeGainX*Time-RWPositionGainX*(RWPositionX-RWPositionSetpointX)...
    -RWDampeningX*RWVelocityX);
    JointTorqueRWY=Killswitch*GlobalGain*(RWConstantY+RWTimeGainY*Time-RWPositionGainY*(RWPositionY-RWPositionSetpointY)...
    -RWDampeningY*RWVelocityY);
elseif ModelingMode==3
    JointTorqueRWX=HexPolyInputFunction(RWInputXA,RWInputXB,RWInputXC,RWInputXD,RWInputXE,RWInputXF,RWInputXG,Time)*Killswitch;
    JointTorqueRWY=HexPolyInputFunction(RWInputYA,RWInputYB,RWInputYC,RWInputYD,RWInputYE,RWInputYF,RWInputYG,Time)*Killswitch;  
else
    %ZVCF Based Joint Torques. Values are pulled from model workspace and
    %held constant.
    JointTorqueRWX=ZVCFRWTorqueX;
    JointTorqueRWY=ZVCFRWTorqueY;
end

% Create a global vector of the joint torque inputs
RWJointTorqueInputLocal=cat(1,JointTorqueRWX,JointTorqueRWY,0);
RWJointTorqueInputGlobal=RWLocaltoGlobalR*RWJointTorqueInputLocal;

% Compare total torque measured to input torques applied to see the
% constraint torque

RWConstraintTorque=RWTorqueGlobal-RWJointTorqueInputGlobal;

% %%%%%%%%%%%%%%%%%%%%%%%%%%%%%%%%%%%%%%%%%%%
% % Kinematic Input Selection and Calculation
% %%%%%%%%%%%%%%%%%%%%%%%%%%%%%%%%%%%%%%%%%%%

if KinematicMode==0
    % All kinematic values set to zero.
    RWPositionInputX=0;
    RWPositionInputY=0;
    RWVelocityInputX=0;
    RWVelocityInputY=0;
    RWAccelerationInputX=0;
    RWAccelerationInputY=0;
elseif KinematicMode==1
    % 1st Order Acceleration, 2nd Order Velocity, 3rd Order Position Solution
    PTX=TargetRWPositionX;       
    VTX=TargetRWVelocityX;
    PTY=TargetRWPositionY;
    VTY=TargetRWVelocityY;
    % Define Starting Position and Velocity
    PIX=RWStartPositionX;
    VIX=RWStartVelocityX;
    PIY=RWStartPositionY;
    VIY=RWStartVelocityY;
    AX=3*((VTX+VIX)*TargetImpactTime-2*(PTX-PIX))/TargetImpactTime^3;         % Constant in position equation
    BX=-2*((VTX+2*VIX)*TargetImpactTime-3*(PTX-PIX))/TargetImpactTime^2;         % Constant in position equation
    CX=VIX;         % Starting Velocity at Time Zero
    DX=PIX;         % Starting Position at Time Zero
    AY=3*((VTY+VIY)*TargetImpactTime-2*(PTY-PIY))/TargetImpactTime^3;         % Constant in position equation
    BY=-2*((VTY+2*VIY)*TargetImpactTime-3*(PTY-PIY))/TargetImpactTime^2;         % Constant in position equation
    CY=VIY;         % Starting Velocity at Time Zero
    DY=PIY;         % Starting Position at Time Zero
    % Equation for position as a function of time
    RWPositionInputX=AX*Time^3/3+BX*Time^2/2+CX*Time+DX;
    RWPositionInputY=AY*Time^3/3+BY*Time^2/2+CY*Time+DY;
    RWVelocityInputX=AX*Time^2+BX*Time+CX;
    RWVelocityInputY=AY*Time^2+BY*Time+CY;
    RWAccelerationInputX=2*AX*Time+BX;
    RWAccelerationInputY=2*AY*Time+BY;
elseif KinematicMode==2
    % 2nd Order Acceleration, 3rd Order Velocity, 4th Order Position Solution
    Tt=TargetImpactTime;
    t=Time;
    PoX=RWStartPositionX;
    PoY=RWStartPositionY;
    VoX=RWStartVelocityX;
    VoY=RWStartVelocityY;
    PfX=TargetRWPositionX;
    PfY=TargetRWPositionY;
    VfX=TargetRWVelocityX;
    VfY=TargetRWVelocityY;
    AoX=RWAoX;
    AoY=RWAoY;
    RWPositionInputX=PoX + VoX*t + (AoX*t^2)/2 - (t^3*(4*PoX - 4*PfX + Tt*VfX + 3*Tt*VoX + AoX*Tt^2))/Tt^3 + (t^4*(6*PoX - 6*PfX + 2*Tt*VfX + 4*Tt*VoX + AoX*Tt^2))/(2*Tt^4);
    RWPositionInputY=PoY + VoY*t + (AoY*t^2)/2 - (t^3*(4*PoY - 4*PfY + Tt*VfY + 3*Tt*VoY + AoY*Tt^2))/Tt^3 + (t^4*(6*PoY - 6*PfY + 2*Tt*VfY + 4*Tt*VoY + AoY*Tt^2))/(2*Tt^4);
    RWVelocityInputX=VoX + AoX*t - (3*t^2*(4*PoX - 4*PfX + Tt*VfX + 3*Tt*VoX + AoX*Tt^2))/Tt^3 + (2*t^3*(6*PoX - 6*PfX + 2*Tt*VfX + 4*Tt*VoX + AoX*Tt^2))/Tt^4;
    RWVelocityInputY=VoY + AoY*t - (3*t^2*(4*PoY - 4*PfY + Tt*VfY + 3*Tt*VoY + AoY*Tt^2))/Tt^3 + (2*t^3*(6*PoY - 6*PfY + 2*Tt*VfY + 4*Tt*VoY + AoY*Tt^2))/Tt^4;
    RWAccelerationInputX=AoX + (6*t^2*(6*PoX - 6*PfX + 2*Tt*VfX + 4*Tt*VoX + AoX*Tt^2))/Tt^4 - (6*t*(4*PoX - 4*PfX + Tt*VfX + 3*Tt*VoX + AoX*Tt^2))/Tt^3;
    RWAccelerationInputY=AoY + (6*t^2*(6*PoY - 6*PfY + 2*Tt*VfY + 4*Tt*VoY + AoY*Tt^2))/Tt^4 - (6*t*(4*PoY - 4*PfY + Tt*VfY + 3*Tt*VoY + AoY*Tt^2))/Tt^3;
else
    % 3rd Order Acceleration, 4th Order Velocity, 5th Order Position Solution
    Tt=TargetImpactTime;
    t=Time;
    PoX=RWStartPositionX;
    PoY=RWStartPositionY;
    VoX=RWStartVelocityX;
    VoY=RWStartVelocityY;
    PfX=TargetRWPositionX;
    PfY=TargetRWPositionY;
    VfX=TargetRWVelocityX;
    VfY=TargetRWVelocityY;
    AoX=RWAoX;
    AoY=RWAoY;
    AfX=RWAfX;
    AfY=RWAfY;
    RWPositionInputX=PoX+VoX*t+(AoX*t^2)/2-(t^5*(12*PoX-12*PfX+6*Tt*VfX+6*Tt*VoX-AfX*Tt^2+AoX*Tt^2))/(2*Tt^5)-(t^3*(20*PoX-20*PfX+8*Tt*VfX+12*Tt*VoX-AfX*Tt^2+3*AoX*Tt^2))/(2*Tt^3)+(t^4*(30*PoX-30*PfX+14*Tt*VfX+16*Tt*VoX-2*AfX*Tt^2+3*AoX*Tt^2))/(2*Tt^4);
    RWPositionInputY=PoY+VoY*t+(AoY*t^2)/2-(t^5*(12*PoY-12*PfY+6*Tt*VfY+6*Tt*VoY-AfY*Tt^2+AoY*Tt^2))/(2*Tt^5)-(t^3*(20*PoY-20*PfY+8*Tt*VfY+12*Tt*VoY-AfY*Tt^2+3*AoY*Tt^2))/(2*Tt^3)+(t^4*(30*PoY-30*PfY+14*Tt*VfY+16*Tt*VoY-2*AfY*Tt^2+3*AoY*Tt^2))/(2*Tt^4);  
    RWVelocityInputX=VoX+AoX*t-(5*t^4*(12*PoX-12*PfX+6*Tt*VfX+6*Tt*VoX-AfX*Tt^2+AoX*Tt^2))/(2*Tt^5)-(3*t^2*(20*PoX-20*PfX+8*Tt*VfX+12*Tt*VoX-AfX*Tt^2+3*AoX*Tt^2))/(2*Tt^3)+(2*t^3*(30*PoX-30*PfX+14*Tt*VfX+16*Tt*VoX-2*AfX*Tt^2+3*AoX*Tt^2))/Tt^4;
    RWVelocityInputY=VoY+AoY*t-(5*t^4*(12*PoY-12*PfY+6*Tt*VfY+6*Tt*VoY-AfY*Tt^2+AoY*Tt^2))/(2*Tt^5)-(3*t^2*(20*PoY-20*PfY+8*Tt*VfY+12*Tt*VoY-AfY*Tt^2+3*AoY*Tt^2))/(2*Tt^3)+(2*t^3*(30*PoY-30*PfY+14*Tt*VfY+16*Tt*VoY-2*AfY*Tt^2+3*AoY*Tt^2))/Tt^4;
    RWAccelerationInputX=AoX-(3*t*(20*PoX-20*PfX+8*Tt*VfX+12*Tt*VoX-AfX*Tt^2+3*AoX*Tt^2))/Tt^3-(10*t^3*(12*PoX-12*PfX+6*Tt*VfX+6*Tt*VoX-AfX*Tt^2+AoX*Tt^2))/Tt^5+(6*t^2*(30*PoX-30*PfX+14*Tt*VfX+16*Tt*VoX-2*AfX*Tt^2+3*AoX*Tt^2))/Tt^4;
    RWAccelerationInputY=AoY-(3*t*(20*PoY-20*PfY+8*Tt*VfY+12*Tt*VoY-AfY*Tt^2+3*AoY*Tt^2))/Tt^3-(10*t^3*(12*PoY-12*PfY+6*Tt*VfY+6*Tt*VoY-AfY*Tt^2+AoY*Tt^2))/Tt^5+(6*t^2*(30*PoY-30*PfY+14*Tt*VfY+16*Tt*VoY-2*AfY*Tt^2+3*AoY*Tt^2))/Tt^4;
end

% Calculate Higher Order Derivatives of the Position Outputs
RWJerkX=gradient(RWAccelerationInputX,t);
RWJerkY=gradient(RWAccelerationInputY,t);
RWSnapX=gradient(RWJerkX,t);
RWSnapY=gradient(RWJerkY,t);
RWCrackleX=gradient(RWSnapX,t);
RWCrackleY=gradient(RWSnapY,t);
RWPopX=gradient(RWCrackleX,t);
RWPopY=gradient(RWCrackleY,t);

== matlab function GolfSwing3D_KineticallyDrivenBlockCountStrip/LE Input Function/Left Elbow Input Torque ==
  data: Time input; Killswitch input; JointTorqueLE output; LEPositionInput output; LEInputB parameter; LEPositionSetpoint parameter; GlobalGain parameter; LEDampening parameter; ModelingMode parameter; GlobalPCGain parameter; GlobalVCGain parameter; DampeningGlobalGain parameter; TargetImpactTime parameter; KinematicMode parameter; LEAo parameter; LEStartPosition parameter; LEStartVelocity parameter; LEVCGain parameter; TargetLEVelocity parameter; TargetLEPosition parameter; LEPositionGain parameter; LEInputC parameter; LETimeGain parameter; LEVelocityInput output; LEAccelerationInput output; LEConstant parameter; LEPosition input; LEVelocity input; ZVCFLETorque parameter; LEPCGain parameter; LEInputA parameter; LEAf parameter; LEInputD parameter; LEInputE parameter; LEInputF parameter; LEInputG parameter
function [JointTorqueLE,LEPositionInput,LEVelocityInput,...
    LEAccelerationInput]  = fcn(Time,Killswitch,...
    LEInputB,LEPositionSetpoint,GlobalGain,...
    LEDampening, ModelingMode,GlobalPCGain, GlobalVCGain,...
    DampeningGlobalGain,TargetImpactTime,KinematicMode, LEAo,LEStartPosition,...
    LEStartVelocity,LEVCGain,...
    TargetLEVelocity,TargetLEPosition, ...
    LEPositionGain,LEInputC,...
    LETimeGain, LEConstant, LEPosition,LEVelocity, ZVCFLETorque, LEPCGain, LEInputA,...
    LEAf, LEInputD, LEInputE, LEInputF, LEInputG)

%Tau=Time/TargetImpactTime;
t=Time;

% %%%%%%%%%%%%%%%%%%%%%%%%%%%%%%%%%%%%%%%%%%%
% % Kinetic Input Selection and Calculation
% %%%%%%%%%%%%%%%%%%%%%%%%%%%%%%%%%%%%%%%%%%%

if ModelingMode==0
    % Values are all set to zero.
    JointTorqueLE=0;
elseif ModelingMode==1
    % Control based strategy. Values are based on difference in value
    % between the current state and desired state.
    % LE Joint Rotational Deltas
    DeltaLEPosition=LEPosition-TargetLEPosition;
    DeltaLEVelocity=LEVelocity-TargetLEVelocity;
    % Control Based Strategy
    JointTorqueLE=DeltaLEPosition*LEPCGain*GlobalPCGain-DeltaLEVelocity*LEVCGain*GlobalVCGain-DampeningGlobalGain*LEDampening*LEVelocity;
elseif ModelingMode==2
    % Forward Dynamics Based Strategy. Values are computed based on a
    % polynomial and a combination of dampening and position gained
    % factors.
    JointTorqueLE=Killswitch*GlobalGain*(LEConstant+LETimeGain*Time-LEPositionGain*(LEPosition-LEPositionSetpoint)...
    -LEDampening*LEVelocity);
elseif ModelingMode==3
    JointTorqueLE=HexPolyInputFunction(LEInputA,LEInputB,LEInputC,LEInputD,LEInputE,LEInputF,LEInputG,Time)*Killswitch;
else
    %ZVCF Based Joint Torques. Values are pulled from model workspace and
    %held constant.
    JointTorqueLE=ZVCFLETorque;
end

% %%%%%%%%%%%%%%%%%%%%%%%%%%%%%%%%%%%%%%%%%%%
% % Kinematic Input Selection and Calculation
% %%%%%%%%%%%%%%%%%%%%%%%%%%%%%%%%%%%%%%%%%%%

if KinematicMode==0
    % All kinematic values set to zero.
    LEPositionInput=0;
    LEPositionInputY=0;
    LEVelocityInput=0;
    LEVelocityInputY=0;
    LEAccelerationInput=0;
    LEAccelerationInputY=0;
elseif KinematicMode==1
    % 1st Order Acceleration, 2nd Order Velocity, 3rd Order Position Solution
    PTX=TargetLEPosition;       
    VTX=TargetLEVelocity;
    % Define Starting Position and Velocity
    PIX=LEStartPosition;
    VIX=LEStartVelocity;
    AX=3*((VTX+VIX)*TargetImpactTime-2*(PTX-PIX))/TargetImpactTime^3;         % Constant in position equation
    BX=-2*((VTX+2*VIX)*TargetImpactTime-3*(PTX-PIX))/TargetImpactTime^2;         % Constant in position equation
    CX=VIX;         % Starting Velocity at Time Zero
    DX=PIX;         % Starting Position at Time Zero
    % Equation for position as a function of time
    LEPositionInput=AX*Time^3/3+BX*Time^2/2+CX*Time+DX;
    LEVelocityInput=AX*Time^2+BX*Time+CX;
    LEAccelerationInput=2*AX*Time+BX;
elseif KinematicMode==2
    % 2nd Order Acceleration, 3rd Order Velocity, 4th Order Position Solution
    Tt=TargetImpactTime;
    t=Time;
    PoX=LEStartPosition;
    VoX=LEStartVelocity;
    PfX=TargetLEPosition;
    VfX=TargetLEVelocity;
    AoX=LEAo;
    LEPositionInput=PoX + VoX*t + (AoX*t^2)/2 - (t^3*(4*PoX - 4*PfX + Tt*VfX + 3*Tt*VoX + AoX*Tt^2))/Tt^3 + (t^4*(6*PoX - 6*PfX + 2*Tt*VfX + 4*Tt*VoX + AoX*Tt^2))/(2*Tt^4);
    LEVelocityInput=VoX + AoX*t - (3*t^2*(4*PoX - 4*PfX + Tt*VfX + 3*Tt*VoX + AoX*Tt^2))/Tt^3 + (2*t^3*(6*PoX - 6*PfX + 2*Tt*VfX + 4*Tt*VoX + AoX*Tt^2))/Tt^4;
    LEAccelerationInput=AoX + (6*t^2*(6*PoX - 6*PfX + 2*Tt*VfX + 4*Tt*VoX + AoX*Tt^2))/Tt^4 - (6*t*(4*PoX - 4*PfX + Tt*VfX + 3*Tt*VoX + AoX*Tt^2))/Tt^3;
else
    % 3rd Order Acceleration, 4th Order Velocity, 5th Order Position Solution
    Tt=TargetImpactTime;
    t=Time;
    PoX=LEStartPosition;
    VoX=LEStartVelocity;
    PfX=TargetLEPosition;
    VfX=TargetLEVelocity;
    AoX=LEAo;
    AfX=LEAf;
    LEPositionInput=PoX+VoX*t+(AoX*t^2)/2-(t^5*(12*PoX-12*PfX+6*Tt*VfX+6*Tt*VoX-AfX*Tt^2+AoX*Tt^2))/(2*Tt^5)-(t^3*(20*PoX-20*PfX+8*Tt*VfX+12*Tt*VoX-AfX*Tt^2+3*AoX*Tt^2))/(2*Tt^3)+(t^4*(30*PoX-30*PfX+14*Tt*VfX+16*Tt*VoX-2*AfX*Tt^2+3*AoX*Tt^2))/(2*Tt^4);
    LEVelocityInput=VoX+AoX*t-(5*t^4*(12*PoX-12*PfX+6*Tt*VfX+6*Tt*VoX-AfX*Tt^2+AoX*Tt^2))/(2*Tt^5)-(3*t^2*(20*PoX-20*PfX+8*Tt*VfX+12*Tt*VoX-AfX*Tt^2+3*AoX*Tt^2))/(2*Tt^3)+(2*t^3*(30*PoX-30*PfX+14*Tt*VfX+16*Tt*VoX-2*AfX*Tt^2+3*AoX*Tt^2))/Tt^4;
    LEAccelerationInput=AoX-(3*t*(20*PoX-20*PfX+8*Tt*VfX+12*Tt*VoX-AfX*Tt^2+3*AoX*Tt^2))/Tt^3-(10*t^3*(12*PoX-12*PfX+6*Tt*VfX+6*Tt*VoX-AfX*Tt^2+AoX*Tt^2))/Tt^5+(6*t^2*(30*PoX-30*PfX+14*Tt*VfX+16*Tt*VoX-2*AfX*Tt^2+3*AoX*Tt^2))/Tt^4;
end

% Calculate Higher Order Derivatives of the Position Outputs
LEJerk=gradient(LEAccelerationInput,t);
LESnap=gradient(LEJerk,t);
LECrackle=gradient(LESnap,t);
LEPop=gradient(LECrackle,t);
